simulink model "simulinkDiagramaParte1"  (R2023b)
settings: Solver=VariableStepAuto  StartTime=0.0  StopTime=10.0  RelTol=1e-3
settings Model: Creator=daas0  LastModifiedBy=daas0

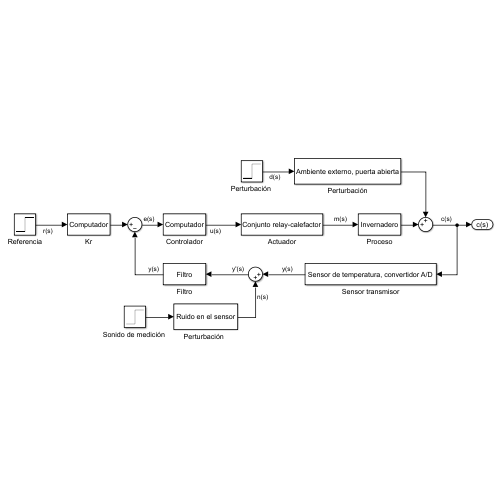
[thumbnail: Simulink's stored preview of the top-level diagram]
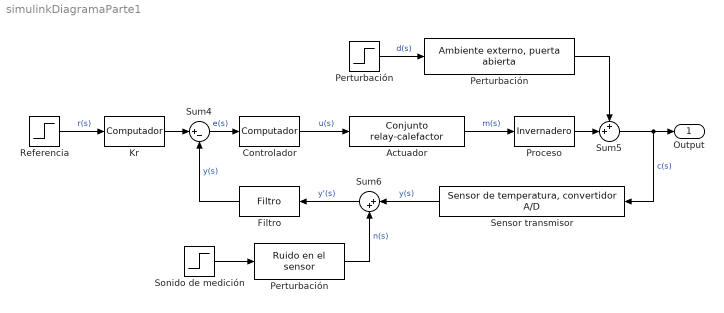
== system simulinkDiagramaParte1 ==
  Actuador : Fcn  Expr=Conjunto relay-calefactor
  Controlador : Fcn  Expr=Computador
  Filtro : Fcn  Expr=Filtro
  Kr : Fcn  Expr=Computador
  Perturbación : Fcn  Expr=Ambiente externo, puerta abierta
  "Perturbación " : Step  Time=16  SampleTime=0
  "Perturbación  " : Fcn  Expr=Ruido en el sensor
  Proceso : Fcn  Expr=Invernadero
  Referencia : Step  SampleTime=0
  Sensor transmisor : Fcn  Expr=Sensor de temperatura, convertidor A/D
  "Sonido de medición " : Step  SampleTime=0
  Sum4 : Sum  Inputs=|+-
  Sum5 : Sum  Inputs=++|
  Sum6 : Sum  Inputs=|++
  Output : Outport
  wires:
  Controlador/1 -> Actuador/1  "u(s)"
  Filtro/1 -> Sum4/2  "y(s)"
  Referencia/1 -> Kr/1  "r(s)"
  Perturbación/1 -> Sum5/1
  "Perturbación "/1 -> Perturbación/1  "d(s)"
  Actuador/1 -> Proceso/1  "m(s)"
  Sensor transmisor/1 -> Sum6/1  "y(s)"
  Proceso/1 -> Sum5/2
  Sum4/1 -> Controlador/1  "e(s)"
  "Sonido de medición "/1 -> "Perturbación  "/1
  Sum6/1 -> Filtro/1  "y'(s)"
  Kr/1 -> Sum4/1
  Sum5/1 -> Output/1, Sensor transmisor/1  "c(s)"
  "Perturbación  "/1 -> Sum6/2  "n(s)"
